simulink model "Greedy_Delay_u"  (R2015a)
settings: Solver=ode5  StartTime=0.0  StopTime=350  FixedStep=0.01  MaxStep=0.01  RelTol=1e-3
values from neighbouring files (symbols this model uses):
  H0 = interp1q(Periodic_Solution(:,1),Periodic_Solution(:,3),Initial_Time-6)    [Gradient_Descent_Controllable_Sleeping.m]
  Periodic_Solution = Periodic_Solution(N:end,:)    [Gradient_Descent_Controllable_Sleeping.m]    (also in Periodic_Solution_PRC_u_1000lux.mat = [0 0.00999999999999 0.02 0.03 0.04 0.05 0.0599999999999 0.06)
  Sleep0 = 0    [Gradient_Descent_Controllable_Sleeping.m]
  theta0 = interp1q(Periodic_Solution(:,1),Periodic_Solution(:,2),Initial_Time-6)    [Gradient_Descent_Controllable_Sleeping.m]
  tol = 0.01    [Gradient_Descent_Controllable_Sleeping.m]
  umax = 0.2208    [Gradient_Descent_Controllable_Sleeping.m]
undefined symbols (not defined in the file or in its folder): f
settings Model: Creator=wangf7  LastModifiedBy=Jiawei Yin
settings OptimizationCC: ExpressionDepthLimit=2147483647
settings DebuggingCC: AlgebraicLoopMsg=none  ArtificialAlgebraicLoopMsg=none  UnderspecifiedInitializationDetection=Classic  MergeDetectMultiDrivingBlocksExec=none  SolverPrmCheckMsg=warning  StateNameClashWarn=warning

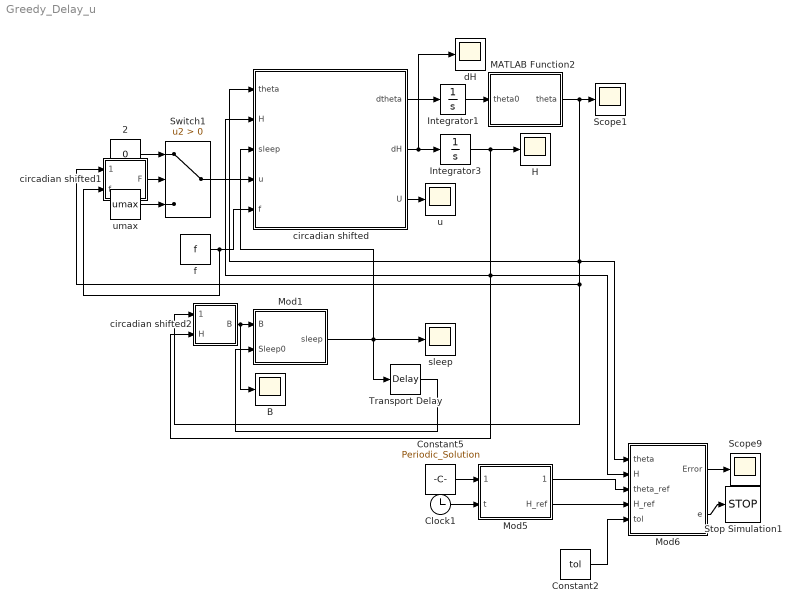
== system Greedy_Delay_u ==
  2 : Constant  Value=0
  B : Scope
      settings: TimeRange=auto  MaxDataPoints=5000000000  SaveName=B  YMin=0.10731  YMax=0.73263  SampleTime=-1  DataFormat=Array
  Clock1 : Clock
  Constant2 : Constant  Value=tol
  Constant5 : Constant  Value=Periodic_Solution
  H : Scope
      settings: TimeRange=auto  MaxDataPoints=5000000000  SaveName=H  YMin=0.01421  YMax=0.71126  SampleTime=-1  DataFormat=Array
  Integrator1 : Integrator  InitialCondition=theta0
  Integrator3 : Integrator  InitialCondition=H0
  MATLAB Function2 : MATLAB Function  TreatAsAtomicUnit=on
      settings: PermitHierarchicalResolution=ParametersOnly
  Mod1 : MATLAB Function  TreatAsAtomicUnit=on
      settings: PermitHierarchicalResolution=ParametersOnly
  Mod5 : MATLAB Function  TreatAsAtomicUnit=on
      settings: PermitHierarchicalResolution=ParametersOnly
  Mod6 : MATLAB Function  TreatAsAtomicUnit=on
      settings: PermitHierarchicalResolution=ParametersOnly
  Scope1 : Scope
      settings: TimeRange=auto  LimitDataPoints=on  MaxDataPoints=5000000000  SaveName=theta  YMin=-0.78492  YMax=7.06682  SampleTime=-1  DataFormat=Array
  Scope9 : Scope
      settings: TimeRange=auto  LimitDataPoints=on  MaxDataPoints=5000000000  SaveName=Error  YMin=-3.9823  YMax=36.90743  SampleTime=-1  DataFormat=Array
  Stop Simulation1 : Stop
  Switch1 : Switch  Criteria=u2 > Threshold
  Transport Delay : TransportDelay  DelayTime=.01  InitialOutput=Sleep0
  circadian shifted : MATLAB Function  TreatAsAtomicUnit=on
      settings: PermitHierarchicalResolution=ParametersOnly
  circadian shifted1 : MATLAB Function  TreatAsAtomicUnit=on
      settings: PermitHierarchicalResolution=ParametersOnly
  circadian shifted2 : MATLAB Function  TreatAsAtomicUnit=on
      settings: PermitHierarchicalResolution=ParametersOnly
  dH : Scope
      settings: TimeRange=auto  MaxDataPoints=5000000000  SaveName=dH  YMin=-0.17777  YMax=0.07567  SampleTime=-1  DataFormat=Array
  f : Constant  Value=f
  sleep : Scope
      settings: TimeRange=auto  MaxDataPoints=5000  SaveName=Sleep  YMin=-0.125  YMax=1.125  SampleTime=-1  DataFormat=Array
  u : Scope
      settings: TimeRange=auto  MaxDataPoints=5000000000  SaveName=u  YMin=-0.0276  YMax=0.2484  SampleTime=-1  DataFormat=Array
  umax : Constant  Value=umax
  wires:
  2/1 -> Switch1/1
  umax/1 -> Switch1/3
  Switch1/1 -> circadian shifted/4(u)
  f/1 -> circadian shifted1/2(f), circadian shifted/5(f)
  circadian shifted/1(dtheta) -> Integrator1/1
  circadian shifted/2(dH) -> dH/1, Integrator3/1
  Integrator1/1 -> MATLAB Function2/1(theta0)
  MATLAB Function2/1(theta) -> Scope1/1, circadian shifted1/1(theta), circadian shifted2/1(theta), Mod6/1(theta), circadian shifted/1(theta)
  Integrator3/1 -> H/1, Mod6/2(H), circadian shifted2/2(H), circadian shifted/2(H)
  circadian shifted2/1(B) -> B/1, Mod1/1(B)
  Mod1/1(sleep) -> Transport Delay/1, sleep/1, circadian shifted/3(sleep)
  Constant5/1 -> Mod5/1(Periodic_Solution)
  Clock1/1 -> Mod5/2(t)
  Mod6/2(e) -> Stop Simulation1/1
  Mod6/1(Error) -> Scope9/1
  Mod5/1(theta_ref) -> Mod6/3(theta_ref)
  Mod5/2(H_ref) -> Mod6/4(H_ref)
  circadian shifted1/1(F) -> Switch1/2
  Constant2/1 -> Mod6/5(tol)
  circadian shifted/3(U) -> u/1
  Transport Delay/1 -> Mod1/2(Sleep0)

== matlab function Greedy_Delay_u/circadian shifted1 ==
  data: theta input; f input; F output
function F = fcn(theta,f)
%#eml
F=interp1q(f(:,1),f(:,2),theta);

== matlab function Greedy_Delay_u/Mod1 ==
  data: sleep output; B input; Sleep0 input
function sleep = fcn(B,Sleep0)
%#codegen
sleep=round(Sleep0);
if B>=0.67
    sleep=1;
elseif B<=0.17
    sleep=0;
end

== matlab function Greedy_Delay_u/circadian shifted ==
  data: theta input; H input; sleep input; u input; dtheta output; dH output; f input; U output
function [dtheta,dH,U] = fcn(theta,H,sleep,u,f)
%#eml
omega0=2*pi/24.2;
tr=18.2;
td=4.2;
U=(1-sleep)*u;
if round(sleep)==0
    dtheta=omega0+interp1q(f(:,1),f(:,2),theta)*u;
    dH=(1-H)/tr;
else
    dtheta=omega0;
    dH=-H/td;
end

== matlab function Greedy_Delay_u/MATLAB Function2 ==
  data: theta0 input; theta output
function theta  = fcn(theta0)

theta=mod(theta0,2*pi);

== matlab function Greedy_Delay_u/circadian shifted2 ==
  data: theta input; H input; B output
function B = fcn(theta,H)
%#eml
B=H-0.1333*cos(theta);

== matlab function Greedy_Delay_u/Mod5 ==
  data: Periodic_Solution input; theta_ref output; t input; H_ref output
function [theta_ref,H_ref] = fcn(Periodic_Solution,t)
%#codegen
theta_ref=interp1q(Periodic_Solution(:,1),Periodic_Solution(:,2),t);
H_ref=interp1q(Periodic_Solution(:,1),Periodic_Solution(:,3),t);

== matlab function Greedy_Delay_u/Mod6 ==
  data: Error output; theta input; H input; e output; theta_ref input; H_ref input; tol input
function [Error,e] = fcn(theta,H,theta_ref,H_ref,tol)
%#codegen
Error=(H-H_ref)^2+min([(theta-theta_ref)^2,(theta-theta_ref-2*pi)^2,(theta-theta_ref+2*pi)^2]);
e=Error<tol;
